simulink model "closed_loop_example"  (R2019b)
settings: Solver=VariableStepAuto  StartTime=0.0  StopTime=1000  FixedStep=.1  RelTol=1e-3
settings Model: Creator=celit  LastModifiedBy=celit
settings SFSimCC: SimCustomHeaderCode="#include \"mono_src/my_func1.h\""  SimUserSources=mono_src/my_func1.cpp  SimUserIncludeDirs=mono_src  SimParseCustomCode=off  CustomCodeUndefinedFunction=UseInterfaceOnly

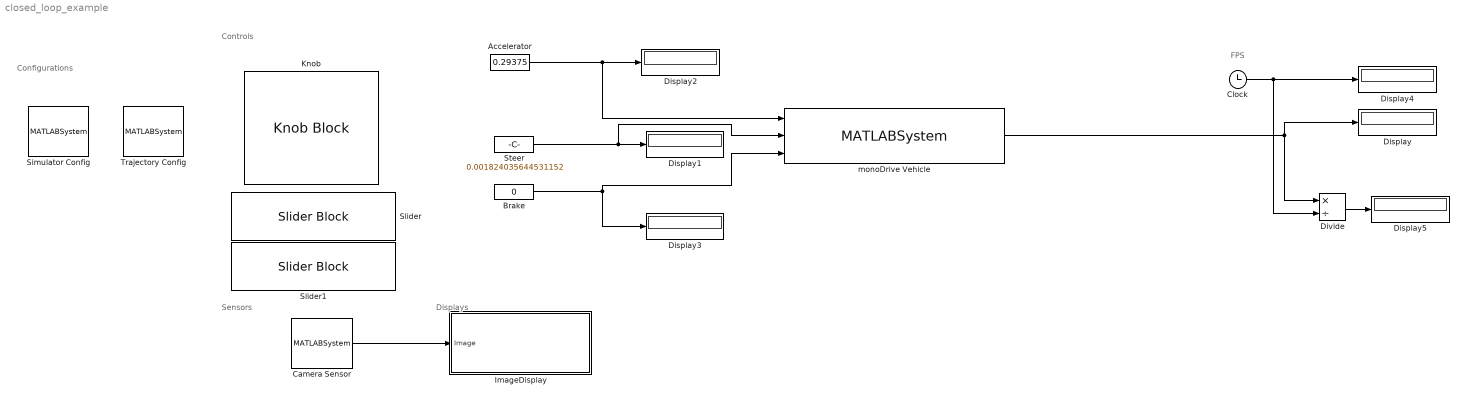
== system closed_loop_example ==
  note: Displays
  note: Controls
  note: Sensors
  note: Configurations
  note: FPS
  Accelerator : Constant  Value=0.29375  OutDataTypeStr=double  SampleTime=-1
  Brake : Constant  Value=0  OutDataTypeStr=double  SampleTime=-1
  Camera Sensor : MATLABSystem  Priority=2  System=Camera  config_path=configurations/camera.json  SampleTime=.0333  OffsetTime=0  TickTime=0.1  SimulateUsing=Interpreted execution
      mask Type: Camera
      mask Display:
      | disp('Camera');
      | port_label('output',1,'y');
  Clock : Clock
  Display{,1..5} (6 alike) : Display
  Divide : Product  Inputs=*/
  ImageDisplay : Subsystem
  Knob : KnobBlock  LabelPosition=Bottom  ScaleMin=-1  ScaleMax=1  TickInterval=.25
  Simulator Config : MATLABSystem  Priority=0  System=Configuration  file_path=configurations/simulator.json  SimulateUsing=Interpreted execution
      mask Type: Configuration
      mask Display: disp('Configuration');
  Slider : SliderBlock  LabelPosition=Bottom  ScaleMax=1  TickInterval=.2
  Slider1 : SliderBlock  LabelPosition=Bottom  ScaleMax=1  TickInterval=.2
  Steer : Constant  Value=0.001824035644531152  SampleTime=-1
  Trajectory Config : MATLABSystem  Priority=1  System=Trajectory  file_path=configurations/trajectories/Close_Loop.json  SimulateUsing=Interpreted execution
      mask Type: Trajectory
      mask Display: disp('Trajectory');
  monoDrive Vehicle : MATLABSystem  Priority=2  System=monoDriveVehicle  SampleTime=.0333  OffsetTime=0  TickTime=.1  SimulateUsing=Interpreted execution
      mask Type: monoDriveVehicle
      mask Display:
      | disp('monoDriveVehicle');
      | port_label('input',1,'forward_amount');
      | port_label('input',2,'right_amount');
      | port_label('input',3,'brake_amount');
      | port_label('output',1,'Count');
  wires:
  Accelerator/1 -> monoDrive Vehicle/1, Display2/1
  Camera Sensor/1 -> ImageDisplay/1(Image)
  monoDrive Vehicle/1 -> Display/1, Divide/1
  Brake/1 -> Display3/1, monoDrive Vehicle/3
  Steer/1 -> monoDrive Vehicle/2, Display1/1
  Clock/1 -> Divide/2, Display4/1
  Divide/1 -> Display5/1

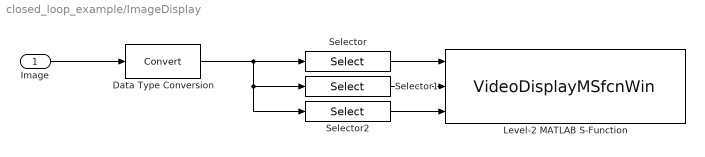
== system closed_loop_example/ImageDisplay ==
  Image : Inport
  Data Type Conversion : DataTypeConversion
  Level-2 MATLAB S-Function : M-S-Function  FunctionName=VideoDisplayMSfcnWin  Parameters=1
  Selector : Selector  NumberOfDimensions=3  InputPortWidth=3  IndexOptions=Select all,Select all,Index vector (dialog)  Indices=[1 3],1,1  OutputSizes=1,1,1
  Selector1 : Selector  NumberOfDimensions=3  InputPortWidth=3  IndexOptions=Select all,Select all,Index vector (dialog)  Indices=[1 3],1,2  OutputSizes=1,1,1
  Selector2 : Selector  NumberOfDimensions=3  InputPortWidth=3  IndexOptions=Select all,Select all,Index vector (dialog)  Indices=[1 3],1,3  OutputSizes=1,1,1
  wires:
  Data Type Conversion/1 -> Selector2/1, Selector1/1, Selector/1
  Image/1 -> Data Type Conversion/1
  Selector1/1 -> Level-2 MATLAB S-Function/2
  Selector2/1 -> Level-2 MATLAB S-Function/3
  Selector/1 -> Level-2 MATLAB S-Function/1
